simulink model "parallel_prediction_and_cost_function_6phase"  (R2022a)
settings: Solver=FixedStepDiscrete  StartTime=0.0  StopTime=10.0  RelTol=1e-3
undefined symbols (not defined in the file or in its folder): f_c, L_d, L_q, L_x, L_y, p, psi_pm, R_ph
libraries: hdlsllib x5
(part 3 of 3)

== system parallel_prediction_and_cost_function_6phase/Prediction_and_cost_function/Subsystem/Subsystem6 ==
  SampleTime_div_Ld : Inport
  SampleTime_div_Lq : Inport  Port=2
  SampleTime_div_Lx : Inport  Port=3
  SampleTime_div_Ly : Inport  Port=4
  d_phase_voltage_per_switching_state : Inport  Port=5
  q_phase_voltage_per_switching_state : Inport  Port=6
  x_phase_voltage_per_switching_state : Inport  Port=7
  y_phase_voltage_per_switching_state : Inport  Port=8
  id_k : Inport  Port=9
  iq_k : Inport  Port=10
  ix_k : Inport  Port=11
  iy_k : Inport  Port=12
  psiPM : Inport  Port=13
  Lq : Inport  Port=14
  Ld : Inport  Port=15
  Rs : Inport  Port=16
  omega_el : Inport  Port=17
  Add{,1,3..4} (4 alike) : Sum  OutDataTypeStr=single
  Add2 : Sum
  Product{1..2,4..11} (10 alike) : Product  OutDataTypeStr=single
  Product3 : Product  Inputs=3  OutDataTypeStr=single
  Subtract : Sum  Inputs=+-+  OutDataTypeStr=single
  Subtract1 : Sum  Inputs=+--  OutDataTypeStr=single
  Subtract2 : Sum  Inputs=+-  OutDataTypeStr=single
  Subtract3 : Sum  Inputs=+-  OutDataTypeStr=single
  id_10 : Outport
  iq_10 : Outport  Port=2
  ix_10 : Outport  Port=3
  iy_10 : Outport  Port=4
  wires:
  q_phase_voltage_per_switching_state/1 -> Subtract1/1
  omega_el/1 -> Product3/1, Product6/1
  Product5/1 -> Subtract1/2
  iq_k/1 -> Product3/3, Add1/2, Product5/1
  iy_k/1 -> Add4/2, Product11/1
  Add2/1 -> Product6/2
  Lq/1 -> Product3/2
  Subtract2/1 -> Product8/2
  SampleTime_div_Ly/1 -> Product10/1
  Rs/1 -> Product9/2, Product2/2, Product5/2, Product11/2
  Product9/1 -> Subtract2/2
  Product8/1 -> Add3/1
  Product7/1 -> Add2/2
  id_k/1 -> Add/2, Product2/1, Product7/1
  x_phase_voltage_per_switching_state/1 -> Subtract2/1
  Product11/1 -> Subtract3/2
  Product6/1 -> Subtract1/3
  Subtract1/1 -> Product4/2
  Product1/1 -> Add/1
  Product10/1 -> Add4/1
  Product4/1 -> Add1/1
  SampleTime_div_Ld/1 -> Product1/1
  y_phase_voltage_per_switching_state/1 -> Subtract3/1
  Product2/1 -> Subtract/2
  Product3/1 -> Subtract/3
  SampleTime_div_Lq/1 -> Product4/1
  Subtract/1 -> Product1/2
  Subtract3/1 -> Product10/2
  psiPM/1 -> Add2/1
  Ld/1 -> Product7/2
  ix_k/1 -> Add3/2, Product9/1
  SampleTime_div_Lx/1 -> Product8/1
  d_phase_voltage_per_switching_state/1 -> Subtract/1
  Add/1 -> id_10/1
  Add1/1 -> iq_10/1
  Add3/1 -> ix_10/1
  Add4/1 -> iy_10/1

== system parallel_prediction_and_cost_function_6phase/Prediction_and_cost_function/Subsystem/Subsystem7 ==
  SampleTime_div_Ld : Inport
  SampleTime_div_Lq : Inport  Port=2
  SampleTime_div_Lx : Inport  Port=3
  SampleTime_div_Ly : Inport  Port=4
  d_phase_voltage_per_switching_state : Inport  Port=5
  q_phase_voltage_per_switching_state : Inport  Port=6
  x_phase_voltage_per_switching_state : Inport  Port=7
  y_phase_voltage_per_switching_state : Inport  Port=8
  id_k : Inport  Port=9
  iq_k : Inport  Port=10
  ix_k : Inport  Port=11
  iy_k : Inport  Port=12
  psiPM : Inport  Port=13
  Lq : Inport  Port=14
  Ld : Inport  Port=15
  Rs : Inport  Port=16
  omega_el : Inport  Port=17
  Add{,1,3..4} (4 alike) : Sum  OutDataTypeStr=single
  Add2 : Sum
  Product{1..2,4..11} (10 alike) : Product  OutDataTypeStr=single
  Product3 : Product  Inputs=3  OutDataTypeStr=single
  Subtract : Sum  Inputs=+-+  OutDataTypeStr=single
  Subtract1 : Sum  Inputs=+--  OutDataTypeStr=single
  Subtract2 : Sum  Inputs=+-  OutDataTypeStr=single
  Subtract3 : Sum  Inputs=+-  OutDataTypeStr=single
  id_9 : Outport
  iq_9 : Outport  Port=2
  ix_9 : Outport  Port=3
  iy_9 : Outport  Port=4
  wires:
  q_phase_voltage_per_switching_state/1 -> Subtract1/1
  omega_el/1 -> Product3/1, Product6/1
  Product5/1 -> Subtract1/2
  iq_k/1 -> Product3/3, Add1/2, Product5/1
  iy_k/1 -> Add4/2, Product11/1
  Add2/1 -> Product6/2
  Lq/1 -> Product3/2
  Subtract2/1 -> Product8/2
  SampleTime_div_Ly/1 -> Product10/1
  Rs/1 -> Product9/2, Product2/2, Product5/2, Product11/2
  Product9/1 -> Subtract2/2
  Product8/1 -> Add3/1
  Product7/1 -> Add2/2
  id_k/1 -> Add/2, Product2/1, Product7/1
  x_phase_voltage_per_switching_state/1 -> Subtract2/1
  Product11/1 -> Subtract3/2
  Product6/1 -> Subtract1/3
  Subtract1/1 -> Product4/2
  Product1/1 -> Add/1
  Product10/1 -> Add4/1
  Product4/1 -> Add1/1
  SampleTime_div_Ld/1 -> Product1/1
  y_phase_voltage_per_switching_state/1 -> Subtract3/1
  Product2/1 -> Subtract/2
  Product3/1 -> Subtract/3
  SampleTime_div_Lq/1 -> Product4/1
  Subtract/1 -> Product1/2
  Subtract3/1 -> Product10/2
  psiPM/1 -> Add2/1
  Ld/1 -> Product7/2
  ix_k/1 -> Add3/2, Product9/1
  SampleTime_div_Lx/1 -> Product8/1
  d_phase_voltage_per_switching_state/1 -> Subtract/1
  Add/1 -> id_9/1
  Add1/1 -> iq_9/1
  Add3/1 -> ix_9/1
  Add4/1 -> iy_9/1

== system parallel_prediction_and_cost_function_6phase/Prediction_and_cost_function/Subsystem/Subsystem8 ==
  SampleTime_div_Ld : Inport
  SampleTime_div_Lq : Inport  Port=2
  SampleTime_div_Lx : Inport  Port=3
  SampleTime_div_Ly : Inport  Port=4
  d_phase_voltage_per_switching_state : Inport  Port=5
  q_phase_voltage_per_switching_state : Inport  Port=6
  x_phase_voltage_per_switching_state : Inport  Port=7
  y_phase_voltage_per_switching_state : Inport  Port=8
  id_k : Inport  Port=9
  iq_k : Inport  Port=10
  ix_k : Inport  Port=11
  iy_k : Inport  Port=12
  psiPM : Inport  Port=13
  Lq : Inport  Port=14
  Ld : Inport  Port=15
  Rs : Inport  Port=16
  omega_el : Inport  Port=17
  Add{,1,3..4} (4 alike) : Sum  OutDataTypeStr=single
  Add2 : Sum
  Product{1..2,4..11} (10 alike) : Product  OutDataTypeStr=single
  Product3 : Product  Inputs=3  OutDataTypeStr=single
  Subtract : Sum  Inputs=+-+  OutDataTypeStr=single
  Subtract1 : Sum  Inputs=+--  OutDataTypeStr=single
  Subtract2 : Sum  Inputs=+-  OutDataTypeStr=single
  Subtract3 : Sum  Inputs=+-  OutDataTypeStr=single
  id_8 : Outport
  iq_8 : Outport  Port=2
  ix_8 : Outport  Port=3
  iy_8 : Outport  Port=4
  wires:
  q_phase_voltage_per_switching_state/1 -> Subtract1/1
  omega_el/1 -> Product3/1, Product6/1
  Product5/1 -> Subtract1/2
  iq_k/1 -> Product3/3, Add1/2, Product5/1
  iy_k/1 -> Add4/2, Product11/1
  Add2/1 -> Product6/2
  Lq/1 -> Product3/2
  Subtract2/1 -> Product8/2
  SampleTime_div_Ly/1 -> Product10/1
  Rs/1 -> Product9/2, Product2/2, Product5/2, Product11/2
  Product9/1 -> Subtract2/2
  Product8/1 -> Add3/1
  Product7/1 -> Add2/2
  id_k/1 -> Add/2, Product2/1, Product7/1
  x_phase_voltage_per_switching_state/1 -> Subtract2/1
  Product11/1 -> Subtract3/2
  Product6/1 -> Subtract1/3
  Subtract1/1 -> Product4/2
  Product1/1 -> Add/1
  Product10/1 -> Add4/1
  Product4/1 -> Add1/1
  SampleTime_div_Ld/1 -> Product1/1
  y_phase_voltage_per_switching_state/1 -> Subtract3/1
  Product2/1 -> Subtract/2
  Product3/1 -> Subtract/3
  SampleTime_div_Lq/1 -> Product4/1
  Subtract/1 -> Product1/2
  Subtract3/1 -> Product10/2
  psiPM/1 -> Add2/1
  Ld/1 -> Product7/2
  ix_k/1 -> Add3/2, Product9/1
  SampleTime_div_Lx/1 -> Product8/1
  d_phase_voltage_per_switching_state/1 -> Subtract/1
  Add/1 -> id_8/1
  Add1/1 -> iq_8/1
  Add3/1 -> ix_8/1
  Add4/1 -> iy_8/1

== system parallel_prediction_and_cost_function_6phase/Prediction_and_cost_function/Subsystem/Subsystem9 ==
  SampleTime_div_Ld : Inport
  SampleTime_div_Lq : Inport  Port=2
  SampleTime_div_Lx : Inport  Port=3
  SampleTime_div_Ly : Inport  Port=4
  d_phase_voltage_per_switching_state : Inport  Port=5
  q_phase_voltage_per_switching_state : Inport  Port=6
  x_phase_voltage_per_switching_state : Inport  Port=7
  y_phase_voltage_per_switching_state : Inport  Port=8
  id_k : Inport  Port=9
  iq_k : Inport  Port=10
  ix_k : Inport  Port=11
  iy_k : Inport  Port=12
  psiPM : Inport  Port=13
  Lq : Inport  Port=14
  Ld : Inport  Port=15
  Rs : Inport  Port=16
  omega_el : Inport  Port=17
  Add{,1,3..4} (4 alike) : Sum  OutDataTypeStr=single
  Add2 : Sum
  Product{1..2,4..11} (10 alike) : Product  OutDataTypeStr=single
  Product3 : Product  Inputs=3  OutDataTypeStr=single
  Subtract : Sum  Inputs=+-+  OutDataTypeStr=single
  Subtract1 : Sum  Inputs=+--  OutDataTypeStr=single
  Subtract2 : Sum  Inputs=+-  OutDataTypeStr=single
  Subtract3 : Sum  Inputs=+-  OutDataTypeStr=single
  id_7 : Outport
  iq_7 : Outport  Port=2
  ix_7 : Outport  Port=3
  iy_7 : Outport  Port=4
  wires:
  q_phase_voltage_per_switching_state/1 -> Subtract1/1
  omega_el/1 -> Product3/1, Product6/1
  Product5/1 -> Subtract1/2
  iq_k/1 -> Product3/3, Add1/2, Product5/1
  iy_k/1 -> Add4/2, Product11/1
  Add2/1 -> Product6/2
  Lq/1 -> Product3/2
  Subtract2/1 -> Product8/2
  SampleTime_div_Ly/1 -> Product10/1
  Rs/1 -> Product9/2, Product2/2, Product5/2, Product11/2
  Product9/1 -> Subtract2/2
  Product8/1 -> Add3/1
  Product7/1 -> Add2/2
  id_k/1 -> Add/2, Product2/1, Product7/1
  x_phase_voltage_per_switching_state/1 -> Subtract2/1
  Product11/1 -> Subtract3/2
  Product6/1 -> Subtract1/3
  Subtract1/1 -> Product4/2
  Product1/1 -> Add/1
  Product10/1 -> Add4/1
  Product4/1 -> Add1/1
  SampleTime_div_Ld/1 -> Product1/1
  y_phase_voltage_per_switching_state/1 -> Subtract3/1
  Product2/1 -> Subtract/2
  Product3/1 -> Subtract/3
  SampleTime_div_Lq/1 -> Product4/1
  Subtract/1 -> Product1/2
  Subtract3/1 -> Product10/2
  psiPM/1 -> Add2/1
  Ld/1 -> Product7/2
  ix_k/1 -> Add3/2, Product9/1
  SampleTime_div_Lx/1 -> Product8/1
  d_phase_voltage_per_switching_state/1 -> Subtract/1
  Add/1 -> id_7/1
  Add1/1 -> iq_7/1
  Add3/1 -> ix_7/1
  Add4/1 -> iy_7/1
